simulink model "PWMcontrolReal2"  (R2020b)
settings: Solver=VariableStepAuto  StartTime=0.0  StopTime=10.0  RelTol=1e-3
values from neighbouring files (symbols this model uses):
  B = 0.396912508    [funcioT.m]
  J = 0.190764151    [funcioT.m]
  Ka = 2.70653716    [funcioT.m]
  Km = Ka    (= 2.70653716)    [funcioT.m]
  L = 1.5e-3    (= 0.0015)    [funcioT.m]
  R = 4.8    [funcioT.m]
libraries: pid_lib x4, eePwmGenerator x3
settings Model: Creator=Asus  LastModifiedBy=Asus
settings SolverCC: ZeroCrossAlgorithm=Adaptive
settings DebuggingCC: IgnoredZcDiagnostic=none

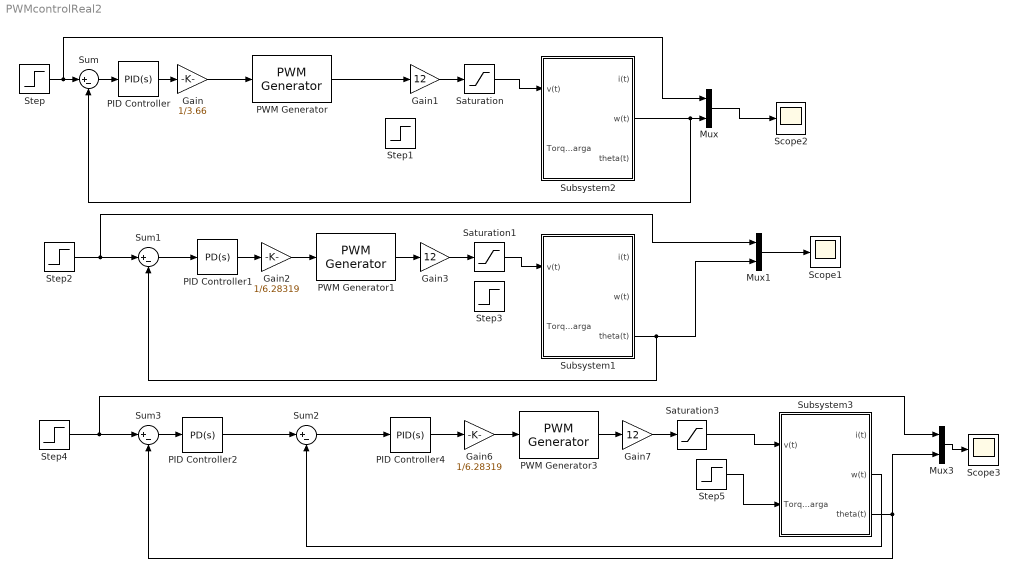
== system PWMcontrolReal2 ==
  Gain : Gain  Gain=1/3.66
  Gain1 : Gain  Gain=12
  Gain2 : Gain  Gain=1/6.28319
  Gain3 : Gain  Gain=12
  Gain6 : Gain  Gain=1/6.28319
  Gain7 : Gain  Gain=12
  Mux : Mux  Inputs=2
  Mux1 : Mux  Inputs=2
  Mux3 : Mux  Inputs=2
  PID Controller : pid_lib/PID Controller  Controller=PID  Form=Parallel  TimeDomain=Continuous-time  UseExternalTs=off  SampleTime=-1  IntegratorMethod=Forward Euler  FilterMethod=Forward Euler  ControllerParametersSource=internal  P=2  I=17.4396027402897  D=0  UseFilter=on  N=100  TunerSelectOption=Transfer Function Based (PID Tuner App)  InitialConditionSource=internal  InitialConditionForIntegrator=0  InitialConditionForFilter=0  DifferentiatorICPrevScaledInput=0  ExternalReset=none  TrackingMode=off  Kt=1  LimitOutput=on  SatLimitsSource=internal  UpperSaturationLimit=3.66  LowerSaturationLimit=0  LinearizeAsGain=on  AntiWindupMode=back-calculation  Kb=1  POutMin=[]  POutMax=[]  IOutMin=[]  IOutMax=[]  DOutMin=[]  DOutMax=[]  NOutMin=[]  NOutMax=[]  SumOutMin=[]  SumOutMax=[]  SaturationOutMin=[]  SaturationOutMax=[]  PParamMin=[]  PParamMax=[]  IParamMin=[]  IParamMax=[]  DParamMin=[]  DParamMax=[]  NParamMin=[]  NParamMax=[]  KbParamMin=[]  KbParamMax=[]  KtParamMin=[]  KtParamMax=[]  KbOutMin=[]  KbOutMax=[]  KtOutMin=[]  KtOutMax=[]  IntegratorOutMin=[]  IntegratorOutMax=[]  FilterOutMin=[]  FilterOutMax=[]  SumI1OutMin=[]  SumI1OutMax=[]  SumI2OutMin=[]  SumI2OutMax=[]  SumI3OutMin=[]  SumI3OutMax=[]  SumI4OutMin=[]  SumI4OutMax=[]  SumDOutMin=[]  SumDOutMax=[]  DifferentiatorOutMin=[]  DifferentiatorOutMax=[]  FilterDiffOutCoefMin=[]  FilterDiffOutCoefMax=[]  ReciprocalOutMin=[]  ReciprocalOutMax=[]  SumDenOutMin=[]  SumDenOutMax=[]  SumNumOutMin=[]  SumNumOutMax=[]  DivideOutMin=[]  DivideOutMax=[]  UdiffTsProdOutMin=[]  UdiffTsProdOutMax=[]  NTsProdOutMin=[]  NTsProdOutMax=[]  UintegralTsProdOutMin=[]  UintegralTsProdOutMax=[]  UngainTsProdOutMin=[]  UngainTsProdOutMax=[]  IntegratorContinuousStateAttributes=''  IntegratorStateMustResolveToSignalObject=off  IntegratorRTWStateStorageClass=Auto  FilterContinuousStateAttributes=''  FilterStateMustResolveToSignalObject=off  FilterRTWStateStorageClass=Auto  ParallelPVariant=InternalParameters  IdealPVariant=Disabled  IVariant=InternalParameters  DVariant=InternalParameters  IntegratorVariant=Continuous  SatVariant=Enabled  AWVariant=BackCalculation  PCopyVariant=Disabled  TRVariant=Disabled  FdbkBlocksVariant=Forward  IdealPFdbkVariant=Disabled  SatFdbkVariant=Disabled  DerivativeFilterVariant=ContFilter  NVariant=InternalParameters  NCopyVariant=Disabled  FilterICVariant=InternalICsFilter  IntegratorICVariant=InternalICs  ExternalResetVariant=Disabled  TRSumVariant=Passthrough  SumFdbkVariant=Disabled  SumVariant=Sum_PID  TsampFilterVariant=InternalTs  TsampNgainVariant=Passthrough  TsampIntegralVariant=Passthrough  ExternalSaturationOutDataTypeStr=Inherit: Same as second input
  PID Controller1 : pid_lib/PID Controller  Controller=PD  Form=Parallel  TimeDomain=Continuous-time  UseExternalTs=off  SampleTime=-1  IntegratorMethod=Forward Euler  FilterMethod=Forward Euler  ControllerParametersSource=internal  P=8  I=10.4332906572305  D=0.27  UseFilter=on  N=4.06515407236639  TunerSelectOption=Transfer Function Based (PID Tuner App)  InitialConditionSource=internal  InitialConditionForIntegrator=0  InitialConditionForFilter=0  DifferentiatorICPrevScaledInput=0  ExternalReset=none  TrackingMode=off  Kt=1  LimitOutput=on  SatLimitsSource=internal  UpperSaturationLimit=1.5708  LowerSaturationLimit=0  LinearizeAsGain=on  AntiWindupMode=clamping  Kb=1  POutMin=[]  POutMax=[]  IOutMin=[]  IOutMax=[]  DOutMin=[]  DOutMax=[]  NOutMin=[]  NOutMax=[]  SumOutMin=[]  SumOutMax=[]  SaturationOutMin=[]  SaturationOutMax=[]  PParamMin=[]  PParamMax=[]  IParamMin=[]  IParamMax=[]  DParamMin=[]  DParamMax=[]  NParamMin=[]  NParamMax=[]  KbParamMin=[]  KbParamMax=[]  KtParamMin=[]  KtParamMax=[]  KbOutMin=[]  KbOutMax=[]  KtOutMin=[]  KtOutMax=[]  IntegratorOutMin=[]  IntegratorOutMax=[]  FilterOutMin=[]  FilterOutMax=[]  SumI1OutMin=[]  SumI1OutMax=[]  SumI2OutMin=[]  SumI2OutMax=[]  SumI3OutMin=[]  SumI3OutMax=[]  SumI4OutMin=[]  SumI4OutMax=[]  SumDOutMin=[]  SumDOutMax=[]  DifferentiatorOutMin=[]  DifferentiatorOutMax=[]  FilterDiffOutCoefMin=[]  FilterDiffOutCoefMax=[]  ReciprocalOutMin=[]  ReciprocalOutMax=[]  SumDenOutMin=[]  SumDenOutMax=[]  SumNumOutMin=[]  SumNumOutMax=[]  DivideOutMin=[]  DivideOutMax=[]  UdiffTsProdOutMin=[]  UdiffTsProdOutMax=[]  NTsProdOutMin=[]  NTsProdOutMax=[]  UintegralTsProdOutMin=[]  UintegralTsProdOutMax=[]  UngainTsProdOutMin=[]  UngainTsProdOutMax=[]  IntegratorContinuousStateAttributes=''  IntegratorStateMustResolveToSignalObject=off  IntegratorRTWStateStorageClass=Auto  FilterContinuousStateAttributes=''  FilterStateMustResolveToSignalObject=off  FilterRTWStateStorageClass=Auto  ParallelPVariant=InternalParameters  IdealPVariant=Disabled  IVariant=Disabled  DVariant=InternalParameters  IntegratorVariant=Disabled  SatVariant=Enabled  AWVariant=Disabled  PCopyVariant=Disabled  TRVariant=Disabled  FdbkBlocksVariant=Forward  IdealPFdbkVariant=Disabled  SatFdbkVariant=Disabled  DerivativeFilterVariant=ContFilter  NVariant=InternalParameters  NCopyVariant=Disabled  FilterICVariant=InternalICsFilter  IntegratorICVariant=Disabled  ExternalResetVariant=Disabled  TRSumVariant=Passthrough  SumFdbkVariant=Disabled  SumVariant=Sum_PD  TsampFilterVariant=InternalTs  TsampNgainVariant=Passthrough  TsampIntegralVariant=Disabled_SignalSpec  ExternalSaturationOutDataTypeStr=Inherit: Same as second input
  PID Controller2 : pid_lib/PID Controller  Controller=PD  Form=Parallel  TimeDomain=Continuous-time  UseExternalTs=off  SampleTime=-1  IntegratorMethod=Forward Euler  FilterMethod=Forward Euler  ControllerParametersSource=internal  P=7  I=34  D=0.9  UseFilter=on  N=3.67190935907782  TunerSelectOption=Transfer Function Based (PID Tuner App)  InitialConditionSource=internal  InitialConditionForIntegrator=0  InitialConditionForFilter=0  DifferentiatorICPrevScaledInput=0  ExternalReset=none  TrackingMode=off  Kt=1  LimitOutput=on  SatLimitsSource=internal  UpperSaturationLimit=1.5708  LowerSaturationLimit=0  LinearizeAsGain=on  AntiWindupMode=clamping  Kb=1  POutMin=[]  POutMax=[]  IOutMin=[]  IOutMax=[]  DOutMin=[]  DOutMax=[]  NOutMin=[]  NOutMax=[]  SumOutMin=[]  SumOutMax=[]  SaturationOutMin=[]  SaturationOutMax=[]  PParamMin=[]  PParamMax=[]  IParamMin=[]  IParamMax=[]  DParamMin=[]  DParamMax=[]  NParamMin=[]  NParamMax=[]  KbParamMin=[]  KbParamMax=[]  KtParamMin=[]  KtParamMax=[]  KbOutMin=[]  KbOutMax=[]  KtOutMin=[]  KtOutMax=[]  IntegratorOutMin=[]  IntegratorOutMax=[]  FilterOutMin=[]  FilterOutMax=[]  SumI1OutMin=[]  SumI1OutMax=[]  SumI2OutMin=[]  SumI2OutMax=[]  SumI3OutMin=[]  SumI3OutMax=[]  SumI4OutMin=[]  SumI4OutMax=[]  SumDOutMin=[]  SumDOutMax=[]  DifferentiatorOutMin=[]  DifferentiatorOutMax=[]  FilterDiffOutCoefMin=[]  FilterDiffOutCoefMax=[]  ReciprocalOutMin=[]  ReciprocalOutMax=[]  SumDenOutMin=[]  SumDenOutMax=[]  SumNumOutMin=[]  SumNumOutMax=[]  DivideOutMin=[]  DivideOutMax=[]  UdiffTsProdOutMin=[]  UdiffTsProdOutMax=[]  NTsProdOutMin=[]  NTsProdOutMax=[]  UintegralTsProdOutMin=[]  UintegralTsProdOutMax=[]  UngainTsProdOutMin=[]  UngainTsProdOutMax=[]  IntegratorContinuousStateAttributes=''  IntegratorStateMustResolveToSignalObject=off  IntegratorRTWStateStorageClass=Auto  FilterContinuousStateAttributes=''  FilterStateMustResolveToSignalObject=off  FilterRTWStateStorageClass=Auto  ParallelPVariant=InternalParameters  IdealPVariant=Disabled  IVariant=Disabled  DVariant=InternalParameters  IntegratorVariant=Disabled  SatVariant=Enabled  AWVariant=Disabled  PCopyVariant=Disabled  TRVariant=Disabled  FdbkBlocksVariant=Forward  IdealPFdbkVariant=Disabled  SatFdbkVariant=Disabled  DerivativeFilterVariant=ContFilter  NVariant=InternalParameters  NCopyVariant=Disabled  FilterICVariant=InternalICsFilter  IntegratorICVariant=Disabled  ExternalResetVariant=Disabled  TRSumVariant=Passthrough  SumFdbkVariant=Disabled  SumVariant=Sum_PD  TsampFilterVariant=InternalTs  TsampNgainVariant=Passthrough  TsampIntegralVariant=Disabled_SignalSpec  ExternalSaturationOutDataTypeStr=Inherit: Same as second input
  PID Controller4 : pid_lib/PID Controller  Controller=PID  Form=Parallel  TimeDomain=Continuous-time  UseExternalTs=off  SampleTime=-1  IntegratorMethod=Forward Euler  FilterMethod=Forward Euler  ControllerParametersSource=internal  P=2  I=17.4396027402897  D=0  UseFilter=on  N=100  TunerSelectOption=Transfer Function Based (PID Tuner App)  InitialConditionSource=internal  InitialConditionForIntegrator=0  InitialConditionForFilter=0  DifferentiatorICPrevScaledInput=0  ExternalReset=none  TrackingMode=off  Kt=1  LimitOutput=on  SatLimitsSource=internal  UpperSaturationLimit=3.66  LowerSaturationLimit=0  LinearizeAsGain=on  AntiWindupMode=back-calculation  Kb=1  POutMin=[]  POutMax=[]  IOutMin=[]  IOutMax=[]  DOutMin=[]  DOutMax=[]  NOutMin=[]  NOutMax=[]  SumOutMin=[]  SumOutMax=[]  SaturationOutMin=[]  SaturationOutMax=[]  PParamMin=[]  PParamMax=[]  IParamMin=[]  IParamMax=[]  DParamMin=[]  DParamMax=[]  NParamMin=[]  NParamMax=[]  KbParamMin=[]  KbParamMax=[]  KtParamMin=[]  KtParamMax=[]  KbOutMin=[]  KbOutMax=[]  KtOutMin=[]  KtOutMax=[]  IntegratorOutMin=[]  IntegratorOutMax=[]  FilterOutMin=[]  FilterOutMax=[]  SumI1OutMin=[]  SumI1OutMax=[]  SumI2OutMin=[]  SumI2OutMax=[]  SumI3OutMin=[]  SumI3OutMax=[]  SumI4OutMin=[]  SumI4OutMax=[]  SumDOutMin=[]  SumDOutMax=[]  DifferentiatorOutMin=[]  DifferentiatorOutMax=[]  FilterDiffOutCoefMin=[]  FilterDiffOutCoefMax=[]  ReciprocalOutMin=[]  ReciprocalOutMax=[]  SumDenOutMin=[]  SumDenOutMax=[]  SumNumOutMin=[]  SumNumOutMax=[]  DivideOutMin=[]  DivideOutMax=[]  UdiffTsProdOutMin=[]  UdiffTsProdOutMax=[]  NTsProdOutMin=[]  NTsProdOutMax=[]  UintegralTsProdOutMin=[]  UintegralTsProdOutMax=[]  UngainTsProdOutMin=[]  UngainTsProdOutMax=[]  IntegratorContinuousStateAttributes=''  IntegratorStateMustResolveToSignalObject=off  IntegratorRTWStateStorageClass=Auto  FilterContinuousStateAttributes=''  FilterStateMustResolveToSignalObject=off  FilterRTWStateStorageClass=Auto  ParallelPVariant=InternalParameters  IdealPVariant=Disabled  IVariant=InternalParameters  DVariant=InternalParameters  IntegratorVariant=Continuous  SatVariant=Enabled  AWVariant=BackCalculation  PCopyVariant=Disabled  TRVariant=Disabled  FdbkBlocksVariant=Forward  IdealPFdbkVariant=Disabled  SatFdbkVariant=Disabled  DerivativeFilterVariant=ContFilter  NVariant=InternalParameters  NCopyVariant=Disabled  FilterICVariant=InternalICsFilter  IntegratorICVariant=InternalICs  ExternalResetVariant=Disabled  TRSumVariant=Passthrough  SumFdbkVariant=Disabled  SumVariant=Sum_PID  TsampFilterVariant=InternalTs  TsampNgainVariant=Passthrough  TsampIntegralVariant=Passthrough  ExternalSaturationOutDataTypeStr=Inherit: Same as second input
  PWM Generator : eePwmGenerator/PWM Generator  CarrCount=Up  Tper=0.005  Ts=1.6e-5
  PWM Generator1 : eePwmGenerator/PWM Generator  CarrCount=Up  Tper=0.005  Ts=1.6e-5
  PWM Generator3 : eePwmGenerator/PWM Generator  CarrCount=Up  Tper=0.005  Ts=1.6e-5
  Saturation : Saturate  UpperLimit=12  LowerLimit=0
  Saturation1 : Saturate  UpperLimit=12  LowerLimit=0
  Saturation3 : Saturate  UpperLimit=12  LowerLimit=0
  Scope1 : Scope
  Scope2 : Scope
  Scope3 : Scope
  Step : Step  Time=0.5  After=3.507  SampleTime=0
  Step1 : Step  After=0.1  SampleTime=0
  Step2 : Step  Time=0.5  After=0.588  SampleTime=0
  Step3 : Step  After=0.1  SampleTime=0
  Step4 : Step  Time=0.5  After=0.588  SampleTime=0
  Step5 : Step  After=0.1  SampleTime=0
  Subsystem1 : Subsystem
  Subsystem2 : Subsystem
  Subsystem3 : Subsystem
  Sum{,1..3} (4 alike) : Sum  Inputs=|+-
  wires:
  Gain1/1 -> Saturation/1
  PID Controller/1 -> Gain/1
  PWM Generator/1 -> Gain1/1
  Gain/1 -> PWM Generator/1
  Saturation/1 -> Subsystem2/1(v(t))
  Step/1 -> Mux/1, Sum/1
  Sum/1 -> PID Controller/1
  Mux/1 -> Scope2/1
  Subsystem2/2(w(t)) -> Sum/2, Mux/2
  Step2/1 -> Mux1/1, Sum1/1
  Saturation1/1 -> Subsystem1/1(v(t))
  Sum1/1 -> PID Controller1/1
  Gain3/1 -> Saturation1/1
  Gain2/1 -> PWM Generator1/1
  PWM Generator1/1 -> Gain3/1
  PID Controller1/1 -> Gain2/1
  Mux1/1 -> Scope1/1
  Subsystem1/3(theta(t)) -> Mux1/2, Sum1/2
  Sum2/1 -> PID Controller4/1
  Saturation3/1 -> Subsystem3/1(v(t))
  Gain7/1 -> Saturation3/1
  PWM Generator3/1 -> Gain7/1
  Gain6/1 -> PWM Generator3/1
  Sum3/1 -> PID Controller2/1
  Subsystem3/3(theta(t)) -> Sum3/2, Mux3/2
  Step4/1 -> Mux3/1, Sum3/1
  PID Controller2/1 -> Sum2/1
  PID Controller4/1 -> Gain6/1
  Subsystem3/2(w(t)) -> Sum2/2
  Mux3/1 -> Scope3/1
  Step5/1 -> Subsystem3/2(Torque Carga)

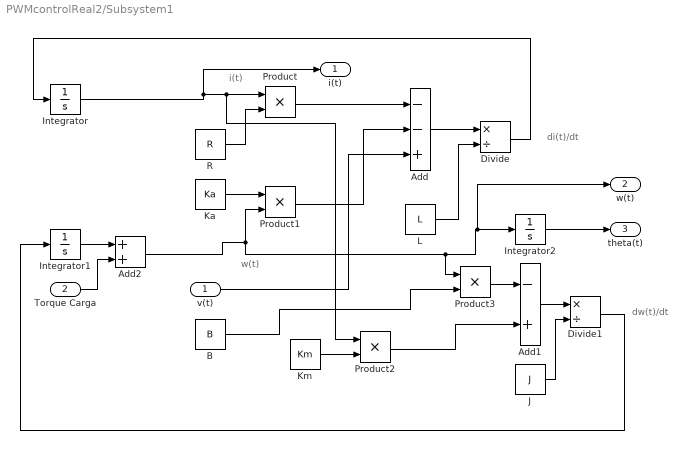
== system PWMcontrolReal2/Subsystem1 ==
  note: i(t)
  note: w(t)
  note: di(t)/dt
  note: dw(t)/dt
  v(t) : Inport
  Torque Carga : Inport  Port=2
  Add : Sum  Inputs=--+
  Add1 : Sum  Inputs=-+
  Add2 : Sum
  B : Constant  Value=B
  Divide : Product  Inputs=*/
  Divide1 : Product  Inputs=*/
  Integrator : Integrator
  Integrator1 : Integrator
  Integrator2 : Integrator
  J : Constant  Value=J
  Ka : Constant  Value=Ka
  Km : Constant  Value=Km
  L : Constant  Value=L
  Product{,1..3} (4 alike) : Product
  R : Constant  Value=R
  i(t) : Outport  VectorParamsAs1DForOutWhenUnconnected=off
  w(t) : Outport  Port=2  VectorParamsAs1DForOutWhenUnconnected=off
  theta(t) : Outport  Port=3  VectorParamsAs1DForOutWhenUnconnected=off
  wires:
  v(t)/1 -> Add/3
  Divide1/1 -> Integrator1/1
  Product1/1 -> Add/2
  Product/1 -> Add/1
  Divide/1 -> Integrator/1
  Km/1 -> Product2/2
  L/1 -> Divide/2
  Add/1 -> Divide/1
  J/1 -> Divide1/2
  Product2/1 -> Add1/2
  B/1 -> Product3/2
  Integrator2/1 -> theta(t)/1
  Add1/1 -> Divide1/1
  Product3/1 -> Add1/1
  R/1 -> Product/2
  Ka/1 -> Product1/1
  Integrator1/1 -> Add2/1
  Torque Carga/1 -> Add2/2
  Integrator/1 -> i(t)/1, Product2/1, Product/1
  Add2/1 -> Product3/1, w(t)/1, Integrator2/1, Product1/2

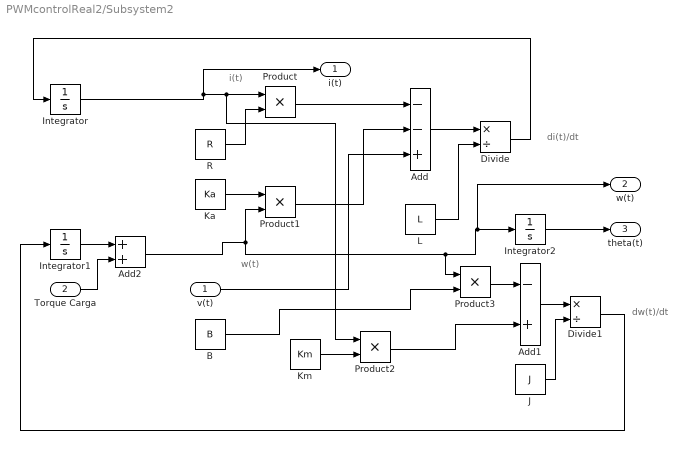
== system PWMcontrolReal2/Subsystem2 ==
  note: i(t)
  note: w(t)
  note: di(t)/dt
  note: dw(t)/dt
  v(t) : Inport
  Torque Carga : Inport  Port=2
  Add : Sum  Inputs=--+
  Add1 : Sum  Inputs=-+
  Add2 : Sum
  B : Constant  Value=B
  Divide : Product  Inputs=*/
  Divide1 : Product  Inputs=*/
  Integrator : Integrator
  Integrator1 : Integrator
  Integrator2 : Integrator
  J : Constant  Value=J
  Ka : Constant  Value=Ka
  Km : Constant  Value=Km
  L : Constant  Value=L
  Product{,1..3} (4 alike) : Product
  R : Constant  Value=R
  i(t) : Outport  VectorParamsAs1DForOutWhenUnconnected=off
  w(t) : Outport  Port=2  VectorParamsAs1DForOutWhenUnconnected=off
  theta(t) : Outport  Port=3  VectorParamsAs1DForOutWhenUnconnected=off
  wires:
  v(t)/1 -> Add/3
  Divide1/1 -> Integrator1/1
  Product1/1 -> Add/2
  Product/1 -> Add/1
  Divide/1 -> Integrator/1
  Km/1 -> Product2/2
  L/1 -> Divide/2
  Add/1 -> Divide/1
  J/1 -> Divide1/2
  Product2/1 -> Add1/2
  B/1 -> Product3/2
  Integrator2/1 -> theta(t)/1
  Add1/1 -> Divide1/1
  Product3/1 -> Add1/1
  R/1 -> Product/2
  Ka/1 -> Product1/1
  Integrator1/1 -> Add2/1
  Torque Carga/1 -> Add2/2
  Integrator/1 -> i(t)/1, Product2/1, Product/1
  Add2/1 -> Product3/1, w(t)/1, Integrator2/1, Product1/2

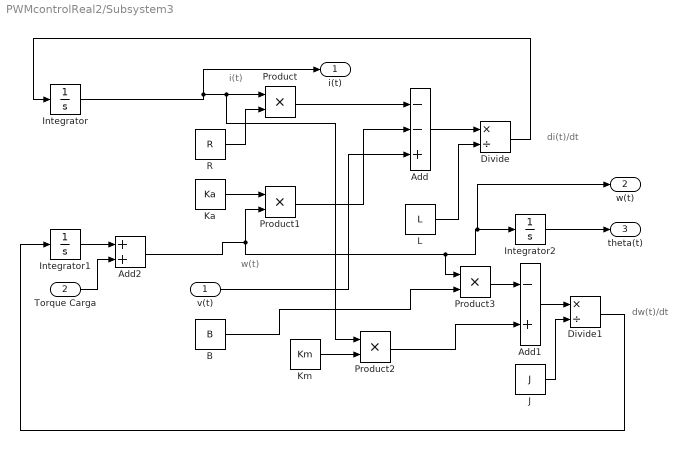
== system PWMcontrolReal2/Subsystem3 ==
  note: i(t)
  note: w(t)
  note: di(t)/dt
  note: dw(t)/dt
  v(t) : Inport
  Torque Carga : Inport  Port=2
  Add : Sum  Inputs=--+
  Add1 : Sum  Inputs=-+
  Add2 : Sum
  B : Constant  Value=B
  Divide : Product  Inputs=*/
  Divide1 : Product  Inputs=*/
  Integrator : Integrator
  Integrator1 : Integrator
  Integrator2 : Integrator
  J : Constant  Value=J
  Ka : Constant  Value=Ka
  Km : Constant  Value=Km
  L : Constant  Value=L
  Product{,1..3} (4 alike) : Product
  R : Constant  Value=R
  i(t) : Outport  VectorParamsAs1DForOutWhenUnconnected=off
  w(t) : Outport  Port=2  VectorParamsAs1DForOutWhenUnconnected=off
  theta(t) : Outport  Port=3  VectorParamsAs1DForOutWhenUnconnected=off
  wires:
  v(t)/1 -> Add/3
  Divide1/1 -> Integrator1/1
  Product1/1 -> Add/2
  Product/1 -> Add/1
  Divide/1 -> Integrator/1
  Km/1 -> Product2/2
  L/1 -> Divide/2
  Add/1 -> Divide/1
  J/1 -> Divide1/2
  Product2/1 -> Add1/2
  B/1 -> Product3/2
  Integrator2/1 -> theta(t)/1
  Add1/1 -> Divide1/1
  Product3/1 -> Add1/1
  R/1 -> Product/2
  Ka/1 -> Product1/1
  Integrator1/1 -> Add2/1
  Torque Carga/1 -> Add2/2
  Integrator/1 -> i(t)/1, Product2/1, Product/1
  Add2/1 -> Product3/1, w(t)/1, Integrator2/1, Product1/2
